simulink model "clik_phi_inverse"  (R2022b)
settings: Solver=ode1  StartTime=0.0  StopTime=4  FixedStep=0.001  RelTol=1e-3
undefined symbols (not defined in the file or in its folder): DiscIntNeverNeededParam, q0, Tc
settings Model: Creator=Xp  LastModifiedBy=CHINMAY PRASHANTH
settings SolverCC: AlgebraicLoopSolver=TrustRegion
settings DataIOCC: LimitDataPoints=on  SaveFormat=Array  SignalLoggingSaveFormat=ModelDataLogs  ReturnWorkspaceOutputs=off
settings OptimizationCC: ExpressionDepthLimit=2147483647  InitFltsAndDblsToZero=on  LifeSpan=inf
settings DebuggingCC: SaveWithParameterizedLinksMsg=none  UnderspecifiedInitializationDetection=Classic  MergeDetectMultiDrivingBlocksExec=none  SolverPrmCheckMsg=warning  MultiTaskDSMMsg=warning  MultiTaskCondExecSysMsg=none  FcnCallInpInsideContextMsg=warning  UnconnectedInputMsg=warning  UnconnectedOutputMsg=warning  UnconnectedLineMsg=warning  StateNameClashWarn=warning  SFUnexpectedBacktrackingDiag=warning  SFNoUnconditionalDefaultTransitionDiag=warning  SFExecutionAtInitializationDiag=none  SFMachineParentedDataDiag=warning  ArithmeticOperatorsInVariantConditions=warning
settings HardwareCC: ProdBitPerPointer=32  ProdBitPerSizeT=32  ProdBitPerPtrDiffT=32  ProdLargestAtomicFloat=None  ProdIntDivRoundTo=Undefined  ProdEndianess=Unspecified  ProdWordSize=32  ProdHWDeviceType=32-bit Generic
settings ModelReferenceCC: EnableRefExpFcnMdlSchedulingChecks=on  PropagateSignalLabelsOutOfModel=off
settings SFSimCC: CustomCodeUndefinedFunction=UseInterfaceOnly
settings RTWCC: DLArmComputeVersion=19.05
settings CodeAppCC: StateflowObjectComments=on
settings GRTTargetCC: TargetLangStandard=C89/C90 (ANSI)  CombineOutputUpdateFcns=off  GRTInterface=on
settings ConfigComp: CovMetricSettings=dw  CovSaveCumulativeToWorkspaceVar=on  CovSaveSingleToWorkspaceVar=on

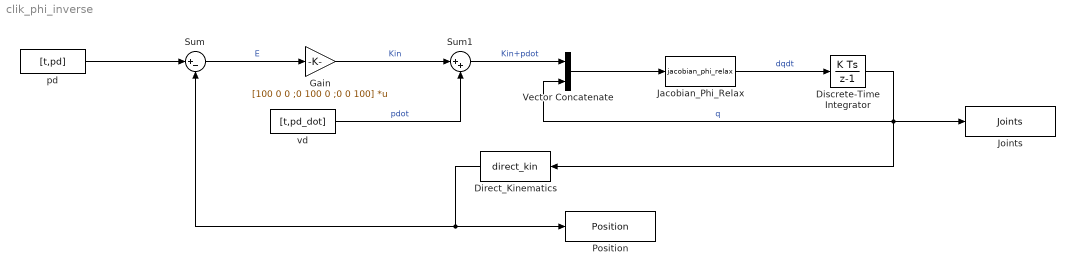
== system clik_phi_inverse ==
  Direct_Kinematics : MATLABFcn  MATLABFcn=direct_kin  OutputDimensions=3  OutputSignalType=real
  Discrete-Time Integrator : DiscreteIntegrator  InitialCondition=q0  SampleTime=Tc  ICPrevOutput=DiscIntNeverNeededParam  ICPrevScaledInput=DiscIntNeverNeededParam
  Gain : Gain  Gain=[100 0 0 ;0 100 0 ;0 0 100]  Multiplication=Matrix(K*u)
  Jacobian_Phi_Relax : MATLABFcn  MATLABFcn=jacobian_phi_relax  OutputSignalType=real
  Joints : ToWorkspace  VariableName=Joints  SampleTime=-1
  Position : ToWorkspace  VariableName=Position  SampleTime=-1
  Sum : Sum  Inputs=|+-
  Sum1 : Sum  Inputs=|++
  Vector Concatenate : Concatenate
  pd : FromWorkspace  VariableName=[t,pd]
  vd : FromWorkspace  VariableName=[t,pd_dot]  SampleTime=Tc
  wires:
  Direct_Kinematics/1 -> Sum/2, Position/1
  Sum/1 -> Gain/1  "E"
  Jacobian_Phi_Relax/1 -> Discrete-Time Integrator/1  "dqdt"
  Discrete-Time Integrator/1 -> Direct_Kinematics/1, Vector Concatenate/2, Joints/1  "q"
  pd/1 -> Sum/1
  Sum1/1 -> Vector Concatenate/1  "Kin+pdot"
  Vector Concatenate/1 -> Jacobian_Phi_Relax/1
  vd/1 -> Sum1/2  "pdot"
  Gain/1 -> Sum1/1  "Kin"
